simulink model "vox_ebersmoll"  (R2023b)
settings: Solver=ode1be  StartTime=0.0  StopTime=stop_time  FixedStep=Ts  RelTol=1e-3
values from neighbouring files (symbols this model uses):
  alpha_f = 236/(236+1)    (= 0.995780590717)    [dataset_generator.m]    (also in groundtruth_generator.m)
  alpha_r = 5.774/(5.774+1)    (= 0.852376734573)    [dataset_generator.m]    (also in groundtruth_generator.m)
  Is1 = 33.58e-15    (= 3.358e-14)    [dataset_generator.m]    (also in groundtruth_generator.m)
  Is2 = 33.58e-15    (= 3.358e-14)    [dataset_generator.m]    (also in groundtruth_generator.m)
  Rp1 = 1e11    (= 100000000000)    [dataset_generator.m]    (also in groundtruth_generator.m)
  Rp2 = 1e8    (= 100000000)    [dataset_generator.m]    (also in groundtruth_generator.m)
  Vt = 25.85e-3    (= 0.02585)    [dataset_generator.m]    (also in groundtruth_generator.m)
libraries: fl_lib x74, nesl_utility x11, ee_lib x1
settings Model: Creator=sebastian  LastModifiedBy=sebastian

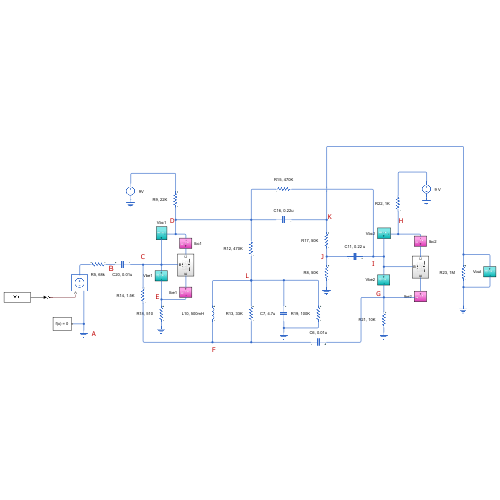
[thumbnail: Simulink's stored preview of the top-level diagram]
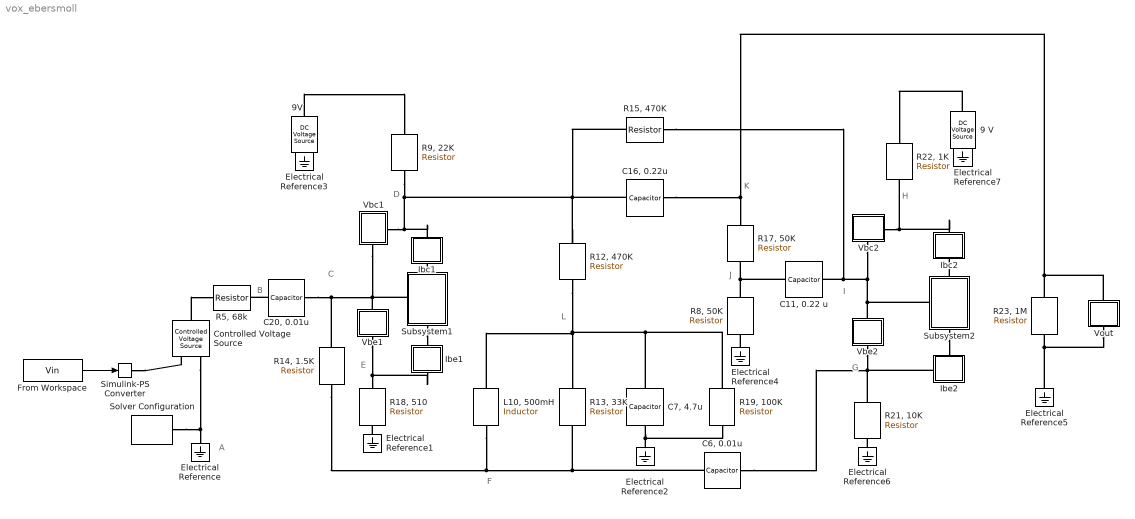
== system vox_ebersmoll ==
  note: I
  note: F
  note: E
  note: C
  note: D
  note: A
  note: B
  note: L
  note: J
  note: K
  note: G
  note: H
  9 V : fl_lib/Electrical/Electrical Sources/DC Voltage Source  v0=9 V
  9V : fl_lib/Electrical/Electrical Sources/DC Voltage Source  v0=9 V
  "C11, 0.22 u" : fl_lib/Electrical/Electrical Elements/Capacitor  c=0.22e-6 F  r=1e-6 Ohm  g=0 1/Ohm  i_specify=off  i_priority=None  i=0 A  i_nominal_specify=off  i_nominal_unit=A  i_nominal_value=1  v_specify=off  v_priority=None  v=0 V  v_nominal_specify=off  v_nominal_unit=V  v_nominal_value=1  vc_specify=off  vc_priority=High  vc=0 V  vc_nominal_specify=off  vc_nominal_unit=V  vc_nominal_value=1
  "C16, 0.22u" : fl_lib/Electrical/Electrical Elements/Capacitor  c=0.22e-6 F  r=1e-6 Ohm  g=0 1/Ohm  i_specify=off  i_priority=None  i=0 A  i_nominal_specify=off  i_nominal_unit=A  i_nominal_value=1  v_specify=off  v_priority=None  v=0 V  v_nominal_specify=off  v_nominal_unit=V  v_nominal_value=1  vc_specify=off  vc_priority=High  vc=0 V  vc_nominal_specify=off  vc_nominal_unit=V  vc_nominal_value=1
  "C20, 0.01u" : fl_lib/Electrical/Electrical Elements/Capacitor  c=0.01e-6 F  r=0 Ohm  g=0 1/Ohm  i_specify=off  i_priority=None  i=0 A  i_nominal_specify=off  i_nominal_unit=A  i_nominal_value=1  v_specify=off  v_priority=None  v=0 V  v_nominal_specify=off  v_nominal_unit=V  v_nominal_value=1  vc_specify=off  vc_priority=High  vc=0 V  vc_nominal_specify=off  vc_nominal_unit=V  vc_nominal_value=1
  "C6, 0.01u" : fl_lib/Electrical/Electrical Elements/Capacitor  c=0.01e-6 F  r=1e-6 Ohm  g=0 1/Ohm  i_specify=off  i_priority=None  i=0 A  i_nominal_specify=off  i_nominal_unit=A  i_nominal_value=1  v_specify=off  v_priority=None  v=0 V  v_nominal_specify=off  v_nominal_unit=V  v_nominal_value=1  vc_specify=off  vc_priority=High  vc=0 V  vc_nominal_specify=off  vc_nominal_unit=V  vc_nominal_value=1
  "C7, 4.7u" : fl_lib/Electrical/Electrical Elements/Capacitor  c=4.7e-6 F  r=1e-6 Ohm  g=0 1/Ohm  i_specify=off  i_priority=None  i=0 A  i_nominal_specify=off  i_nominal_unit=A  i_nominal_value=1  v_specify=off  v_priority=None  v=0 V  v_nominal_specify=off  v_nominal_unit=V  v_nominal_value=1  vc_specify=off  vc_priority=High  vc=0 V  vc_nominal_specify=off  vc_nominal_unit=V  vc_nominal_value=1
  Controlled Voltage Source : fl_lib/Electrical/Electrical Sources/Controlled Voltage Source
  Electrical Reference{,1..7} (8 alike) : fl_lib/Electrical/Electrical Elements/Electrical Reference
  From Workspace : FromWorkspace  VariableName=Vin
  Ibc1 : Subsystem
  Ibc2 : Subsystem
  Ibe1 : Subsystem
  Ibe2 : Subsystem
      settings: PortSchema="{\"entries\":[{\"content\":{\"sides\":[{\"content\":{\"connectorIds\":[\"LConn1\"]},\"type\":\"ConnectorPlacement.EquallySpacedRectSide\",\"uuid\":\"c0c77781-7d19-4b13-84c2-226c323c58f5\"},{\"content\":{\"side\":\"RIGHT\"},\"type\":\"ConnectorPlacement.EquallySpacedRectSide\",\"uuid\":\"c0907413-589c-4dc0-a622-9f77009212b7\"},{\"content\":{\"connectorIds\":[\"LConn2\"],\"side\":\"TOP\"},\"type\":\"ConnectorPlacement.EquallySpacedRectSide\",\"uuid\":\"3bc5d805-3917-4f3d-81f9-d2247414e7c8\"}]},\"type\":\"ConnectorPlacement.EquallySpacedConnector\",\"uuid\":\"4bd7f28c-fe76-4fbf-a473-c2892e027990\"}],\"packageUris\":[\"http://schema.mathworks.com/mf0/Connector/R2020b\"],\"version\":\"1.0\"}"
  "L10, 500mH" : ee_lib/Passive/Inductor  l=0.5 H  enable_L_tol=ee.enum.toleranceApplication.none  L_tol=20  tol_distribution=ee.enum.toleranceDistribution.uniform  nSigma=4  r=0 Ohm  g=1e-9 1/Ohm  enable_operating_limits=ee.enum.enable.no  operating_limit_action=ee.enum.passive.reportOpLim.warn  max_working_current=1 A  power_rating=1 W  enable_faults=ee.enum.enable.no  fault_action=simscape.enum.assert.action.none  lambdaPercent=50  k_faulted=0.9999  turnsShort=ee.enum.passive.inductor.turnsShortOption.no  openCct=ee.enum.enable.no  groundShort=ee.enum.passive.inductor.groundShortOption.no  groundShortG=0 1/Ohm  tau_fault=1e-3 s  fault_trigger=ee.enum.faults.faultTrigger.temporal  t_fault=1 s  max_permissible_voltage=100 V  n_fail_on_voltage=1  max_permissible_current=1 A  t_fail_on_current=1 s  i_L_specify=off  i_L_priority=High  i_L=0 A  i_L_nominal_specify=off  i_L_nominal_unit=A  i_L_nominal_value=1
  "R12, 470K" : fl_lib/Electrical/Electrical Elements/Resistor  R=470e3 Ohm  i_specify=off  i_priority=None  i=0 A  i_nominal_specify=off  i_nominal_unit=A  i_nominal_value=1  v_specify=off  v_priority=None  v=0 V  v_nominal_specify=off  v_nominal_unit=V  v_nominal_value=1
  "R13, 33K" : fl_lib/Electrical/Electrical Elements/Resistor  R=33e3 Ohm  i_specify=off  i_priority=None  i=0 A  i_nominal_specify=off  i_nominal_unit=A  i_nominal_value=1  v_specify=off  v_priority=None  v=0 V  v_nominal_specify=off  v_nominal_unit=V  v_nominal_value=1
  "R14, 1.5K" : fl_lib/Electrical/Electrical Elements/Resistor  R=1.5e3 Ohm  i_specify=off  i_priority=None  i=0 A  i_nominal_specify=off  i_nominal_unit=A  i_nominal_value=1  v_specify=off  v_priority=None  v=0 V  v_nominal_specify=off  v_nominal_unit=V  v_nominal_value=1
  "R15, 470K" : fl_lib/Electrical/Electrical Elements/Resistor  R=470e3 Ohm  i_specify=off  i_priority=None  i=0 A  i_nominal_specify=off  i_nominal_unit=A  i_nominal_value=1  v_specify=off  v_priority=None  v=0 V  v_nominal_specify=off  v_nominal_unit=V  v_nominal_value=1
  "R17, 50K" : fl_lib/Electrical/Electrical Elements/Resistor  R=50e3 Ohm  i_specify=off  i_priority=None  i=0 A  i_nominal_specify=off  i_nominal_unit=A  i_nominal_value=1  v_specify=off  v_priority=None  v=0 V  v_nominal_specify=off  v_nominal_unit=V  v_nominal_value=1
  "R18, 510" : fl_lib/Electrical/Electrical Elements/Resistor  R=510 Ohm  i_specify=off  i_priority=None  i=0 A  i_nominal_specify=off  i_nominal_unit=A  i_nominal_value=1  v_specify=off  v_priority=None  v=0 V  v_nominal_specify=off  v_nominal_unit=V  v_nominal_value=1
  "R19, 100K" : fl_lib/Electrical/Electrical Elements/Resistor  R=100e3 Ohm  i_specify=off  i_priority=None  i=0 A  i_nominal_specify=off  i_nominal_unit=A  i_nominal_value=1  v_specify=off  v_priority=None  v=0 V  v_nominal_specify=off  v_nominal_unit=V  v_nominal_value=1
  "R21, 10K" : fl_lib/Electrical/Electrical Elements/Resistor  R=10e3 Ohm  i_specify=off  i_priority=None  i=0 A  i_nominal_specify=off  i_nominal_unit=A  i_nominal_value=1  v_specify=off  v_priority=None  v=0 V  v_nominal_specify=off  v_nominal_unit=V  v_nominal_value=1
  "R22, 1K" : fl_lib/Electrical/Electrical Elements/Resistor  R=1e3 Ohm  i_specify=off  i_priority=None  i=0 A  i_nominal_specify=off  i_nominal_unit=A  i_nominal_value=1  v_specify=off  v_priority=None  v=0 V  v_nominal_specify=off  v_nominal_unit=V  v_nominal_value=1
  "R23, 1M" : fl_lib/Electrical/Electrical Elements/Resistor  R=1e6 Ohm  i_specify=off  i_priority=None  i=0 A  i_nominal_specify=off  i_nominal_unit=A  i_nominal_value=1  v_specify=off  v_priority=None  v=0 V  v_nominal_specify=off  v_nominal_unit=V  v_nominal_value=1
  "R5, 68k" : fl_lib/Electrical/Electrical Elements/Resistor  R=68e3 Ohm  i_specify=off  i_priority=None  i=0 A  i_nominal_specify=off  i_nominal_unit=A  i_nominal_value=1  v_specify=off  v_priority=None  v=0 V  v_nominal_specify=off  v_nominal_unit=V  v_nominal_value=1
  "R8, 50K" : fl_lib/Electrical/Electrical Elements/Resistor  R=50e3 Ohm  i_specify=off  i_priority=None  i=0 A  i_nominal_specify=off  i_nominal_unit=A  i_nominal_value=1  v_specify=off  v_priority=None  v=0 V  v_nominal_specify=off  v_nominal_unit=V  v_nominal_value=1
  "R9, 22K" : fl_lib/Electrical/Electrical Elements/Resistor  R=22e3 Ohm  i_specify=off  i_priority=None  i=0 A  i_nominal_specify=off  i_nominal_unit=A  i_nominal_value=1  v_specify=off  v_priority=None  v=0 V  v_nominal_specify=off  v_nominal_unit=V  v_nominal_value=1
  Simulink-PS Converter : nesl_utility/Simulink-PS Converter  PhysicalDomain=network_engine_domain  SubClassName=ps_input  LeftPortType=input  RightPortType=output  PseudoPeriodic=off  Frequencies=[]  NoiseDistribution=none  NoiseParameters=[]  Unit=1  AffineConversion=off  FilteringAndDerivatives=provide  SimscapeFilterOrder=1  InputFilterTimeConstant=0.001  UdotUserProvided=0
  Solver Configuration : nesl_utility/Solver Configuration  PhysicalDomain=network_engine_domain  SubClassName=solver  LeftPortType=input  RightPortType=generic  Tones=[]  Harmonics=[]  SimulateNoise=off  Profile=off  UseLocalSampling=off  EnableSwitchedLinearOptims=on  FrequencyDomain=off  UseCCode=off  RelTol=0.001  AbsTol=0.001  MinStep=1e-09  ToWorkspace=off  RevertToSquareIcSolve=off  NumHomotopyIterations=100  PhasorMode=off  PhasorModeNumHarmonics=1  ConsistencySolver=NEWTON_XTOL_AFTER_FTOL  IndexReductionMethod=DerivativeReplacement  DoDC=on  ResidualTolerance=1e-09  ConsistencyTolSource=GLOBAL  ConsistencyAbsTol=0.001  ConsistencyRelTol=0.001  ConsistencyTolFactor=0.001  UseLocalSolver=off  LocalSolverChoice=NE_BACKWARD_EULER_ADVANCER  ResolveIndetEquations=on  FunctionEvalNumThread=1  LocalSolverSampleTime=0.001  DoFixedCost=off  MaxNonlinIter=3  MaxModeIter=2  ComputeImpulses=off  ImpulseIterations=2  LinearAlgebra=auto  LinearAlgebraNumThread=0  EquationFormulation=NE_TIME_EF  DelaysMemoryBudget=1024  AutomaticFiltering=on  FilteringTimeConstant=0.001  PartitionStorageMethod=AS_NEEDED  PartitionMemoryBudget=1024  PartitionMethod=ROBUST  MultibodyUseLocalSolver=off  MultibodyLocalSolverChoice=ODE1  MultibodyLocalSolverSampleTime=0.001
  Subsystem1 : Subsystem
      settings: PortSchema="{\"entries\":[{\"content\":{\"sides\":[{\"content\":{\"connectorIds\":[\"LConn1\"]},\"type\":\"ConnectorPlacement.EquallySpacedRectSide\",\"uuid\":\"e7d2ad01-b729-4278-a2af-615928332c77\"},{\"content\":{\"side\":\"RIGHT\"},\"type\":\"ConnectorPlacement.EquallySpacedRectSide\",\"uuid\":\"6c8f5083-1d74-476b-8fc8-74f7e6a90163\"},{\"content\":{\"connectorIds\":[\"LConn2\"],\"side\":\"TOP\"},\"type\":\"ConnectorPlacement.EquallySpacedRectSide\",\"uuid\":\"cf8d2faf-1e25-415e-bca0-3701d5262d4d\"},{\"content\":{\"connectorIds\":[\"RConn1\"],\"side\":\"BOTTOM\"},\"type\":\"ConnectorPlacement.EquallySpacedRectSide\",\"uuid\":\"80ad8aee-c458-4554-96ef-dc25eb201335\"}]},\"type\":\"ConnectorPlacement.EquallySpacedConnector\",\"uuid\":\"23596b54-1579-47cb-b7ec-00e276fa3e81\"}],\"packageUris\":[\"http://schema.mathworks.com/mf0/Connector/R2020b\"],\"version\":\"1.0\"}"
  Subsystem2 : Subsystem
      settings: PortSchema="{\"entries\":[{\"content\":{\"sides\":[{\"content\":{\"connectorIds\":[\"LConn1\"]},\"type\":\"ConnectorPlacement.EquallySpacedRectSide\",\"uuid\":\"e7d2ad01-b729-4278-a2af-615928332c77\"},{\"content\":{\"side\":\"RIGHT\"},\"type\":\"ConnectorPlacement.EquallySpacedRectSide\",\"uuid\":\"6c8f5083-1d74-476b-8fc8-74f7e6a90163\"},{\"content\":{\"connectorIds\":[\"LConn2\"],\"side\":\"TOP\"},\"type\":\"ConnectorPlacement.EquallySpacedRectSide\",\"uuid\":\"cf8d2faf-1e25-415e-bca0-3701d5262d4d\"},{\"content\":{\"connectorIds\":[\"RConn1\"],\"side\":\"BOTTOM\"},\"type\":\"ConnectorPlacement.EquallySpacedRectSide\",\"uuid\":\"80ad8aee-c458-4554-96ef-dc25eb201335\"}]},\"type\":\"ConnectorPlacement.EquallySpacedConnector\",\"uuid\":\"23596b54-1579-47cb-b7ec-00e276fa3e81\"}],\"packageUris\":[\"http://schema.mathworks.com/mf0/Connector/R2020b\"],\"version\":\"1.0\"}"
  Vbc1 : Subsystem
      settings: PortSchema="{\"entries\":[{\"content\":{\"sides\":[{\"content\":{\"connectorIds\":[\"LConn1\"]},\"type\":\"ConnectorPlacement.EquallySpacedRectSide\",\"uuid\":\"7eb44552-7f97-4ce7-929d-c8e8969a6339\"},{\"content\":{\"side\":\"RIGHT\"},\"type\":\"ConnectorPlacement.EquallySpacedRectSide\",\"uuid\":\"ace6a3d5-1573-4a81-b16e-bbe1b3c73136\"},{\"content\":{\"side\":\"TOP\"},\"type\":\"ConnectorPlacement.EquallySpacedRectSide\",\"uuid\":\"f287eb84-5a92-47a0-b0c0-f16ac8f6c1fa\"},{\"content\":{\"connectorIds\":[\"RConn1\"],\"side\":\"BOTTOM\"},\"type\":\"ConnectorPlacement.EquallySpacedRectSide\",\"uuid\":\"ef144dba-d688-4ec6-a3ad-e1b4e02b5e22\"}]},\"type\":\"ConnectorPlacement.EquallySpacedConnector\",\"uuid\":\"265b9e65-e5e0-4894-94ad-1de7b98f8ce0\"}],\"packageUris\":[\"http://schema.mathworks.com/mf0/Connector/R2020b\"],\"version\":\"1.0\"}"
  Vbc2 : Subsystem
      settings: PortSchema="{\"entries\":[{\"content\":{\"sides\":[{\"content\":{},\"type\":\"ConnectorPlacement.EquallySpacedRectSide\",\"uuid\":\"7eb44552-7f97-4ce7-929d-c8e8969a6339\"},{\"content\":{\"connectorIds\":[\"RConn1\"],\"side\":\"RIGHT\"},\"type\":\"ConnectorPlacement.EquallySpacedRectSide\",\"uuid\":\"ace6a3d5-1573-4a81-b16e-bbe1b3c73136\"},{\"content\":{\"side\":\"TOP\"},\"type\":\"ConnectorPlacement.EquallySpacedRectSide\",\"uuid\":\"f287eb84-5a92-47a0-b0c0-f16ac8f6c1fa\"},{\"content\":{\"connectorIds\":[\"RConn2\"],\"side\":\"BOTTOM\"},\"type\":\"ConnectorPlacement.EquallySpacedRectSide\",\"uuid\":\"ef144dba-d688-4ec6-a3ad-e1b4e02b5e22\"}]},\"type\":\"ConnectorPlacement.EquallySpacedConnector\",\"uuid\":\"265b9e65-e5e0-4894-94ad-1de7b98f8ce0\"}],\"packageUris\":[\"http://schema.mathworks.com/mf0/Connector/R2020b\"],\"version\":\"1.0\"}"
  Vbe1 : Subsystem
  Vbe2 : Subsystem
  Vout : Subsystem
  wires:
  From Workspace/1 -> Simulink-PS Converter/1
  connections:
  Solver Configuration/RConn1 -- Controlled Voltage Source/RConn2 -- Electrical Reference/LConn1
  Controlled Voltage Source/LConn1 -- "R5, 68k"/LConn1
  "C20, 0.01u"/LConn1 -- "R5, 68k"/RConn1
  "R9, 22K"/RConn1 -- Vbc1/LConn1 -- Ibc1/RConn1 -- "R15, 470K"/RConn1 -- "R12, 470K"/LConn1 -- "C16, 0.22u"/RConn1
  Electrical Reference3/LConn1 -- 9V/RConn1
  Vbe1/LConn1 -- Vbc1/RConn1 -- "C20, 0.01u"/RConn1 -- "R14, 1.5K"/LConn1 -- Subsystem1/LConn1
  Vbe1/RConn1 -- Ibe1/RConn1 -- "R18, 510"/LConn1
  "R12, 470K"/RConn1 -- "R13, 33K"/LConn1 -- "L10, 500mH"/LConn1 -- "R19, 100K"/LConn1 -- "C7, 4.7u"/LConn1
  "L10, 500mH"/RConn1 -- "R14, 1.5K"/RConn1 -- "C6, 0.01u"/RConn1 -- "R13, 33K"/RConn1
  Electrical Reference2/LConn1 -- "R19, 100K"/RConn1 -- "C7, 4.7u"/RConn1
  "R8, 50K"/LConn1 -- "C11, 0.22 u"/RConn1 -- "R17, 50K"/RConn1
  "C16, 0.22u"/LConn1 -- Vout/LConn1 -- "R23, 1M"/LConn1 -- "R17, 50K"/LConn1
  Electrical Reference4/LConn1 -- "R8, 50K"/RConn1
  "R15, 470K"/LConn1 -- Vbe2/LConn1 -- Subsystem2/LConn1 -- Vbc2/RConn1 -- "C11, 0.22 u"/LConn1
  Electrical Reference5/LConn1 -- Vout/RConn1 -- "R23, 1M"/RConn1
  "C6, 0.01u"/LConn1 -- Ibe2/LConn2 -- "R21, 10K"/LConn1 -- Vbe2/RConn1
  Electrical Reference6/LConn1 -- "R21, 10K"/RConn1
  Vbc2/RConn2 -- Ibc2/RConn1 -- "R22, 1K"/RConn1
  Electrical Reference7/LConn1 -- 9 V/RConn1
  9 V/LConn1 -- "R22, 1K"/LConn1
  Simulink-PS Converter/RConn1 -- Controlled Voltage Source/RConn1
  Subsystem1/RConn1 -- Ibe1/LConn1
  Subsystem1/LConn2 -- Ibc1/LConn1
  Subsystem2/LConn2 -- Ibc2/LConn1
  Subsystem2/RConn1 -- Ibe2/LConn1
  9V/LConn1 -- "R9, 22K"/LConn1
  Electrical Reference1/LConn1 -- "R18, 510"/RConn1

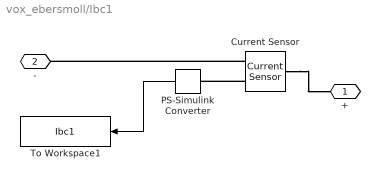
== system vox_ebersmoll/Ibc1 ==
  Current Sensor : fl_lib/Electrical/Electrical Sensors/Current Sensor
  PS-Simulink Converter : nesl_utility/PS-Simulink Converter  PhysicalDomain=network_engine_domain  SubClassName=ps_output  LeftPortType=input  RightPortType=output  PseudoPeriodic=off  Frequencies=[]  VectorFormat=1-D array  Unit=1  AffineConversion=off
  To Workspace1 : ToWorkspace  VariableName=Ibc1  SaveFormat=Timeseries  SampleTime=-1
  + : PMIOPort  Side=Left
  - : PMIOPort  Port=2  Side=Right
  wires:
  PS-Simulink Converter/1 -> To Workspace1/1
  connections:
  Current Sensor/RConn2 -- -/RConn1
  Current Sensor/RConn1 -- PS-Simulink Converter/LConn1
  Current Sensor/LConn1 -- +/RConn1

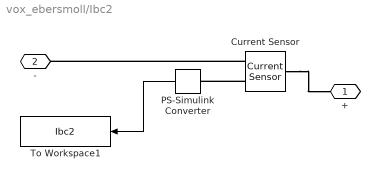
== system vox_ebersmoll/Ibc2 ==
  Current Sensor : fl_lib/Electrical/Electrical Sensors/Current Sensor
  PS-Simulink Converter : nesl_utility/PS-Simulink Converter  PhysicalDomain=network_engine_domain  SubClassName=ps_output  LeftPortType=input  RightPortType=output  PseudoPeriodic=off  Frequencies=[]  VectorFormat=1-D array  Unit=1  AffineConversion=off
  To Workspace1 : ToWorkspace  VariableName=Ibc2  SaveFormat=Timeseries  SampleTime=-1
  + : PMIOPort  Side=Left
  - : PMIOPort  Port=2  Side=Right
  wires:
  PS-Simulink Converter/1 -> To Workspace1/1
  connections:
  Current Sensor/RConn2 -- -/RConn1
  Current Sensor/RConn1 -- PS-Simulink Converter/LConn1
  Current Sensor/LConn1 -- +/RConn1

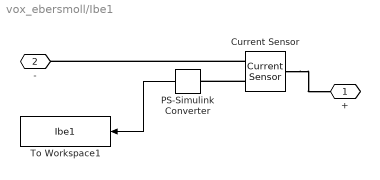
== system vox_ebersmoll/Ibe1 ==
  Current Sensor : fl_lib/Electrical/Electrical Sensors/Current Sensor
  PS-Simulink Converter : nesl_utility/PS-Simulink Converter  PhysicalDomain=network_engine_domain  SubClassName=ps_output  LeftPortType=input  RightPortType=output  PseudoPeriodic=off  Frequencies=[]  VectorFormat=1-D array  Unit=1  AffineConversion=off
  To Workspace1 : ToWorkspace  VariableName=Ibe1  SaveFormat=Timeseries  SampleTime=-1
  + : PMIOPort  Side=Left
  - : PMIOPort  Port=2  Side=Right
  wires:
  PS-Simulink Converter/1 -> To Workspace1/1
  connections:
  Current Sensor/RConn2 -- -/RConn1
  Current Sensor/RConn1 -- PS-Simulink Converter/LConn1
  Current Sensor/LConn1 -- +/RConn1

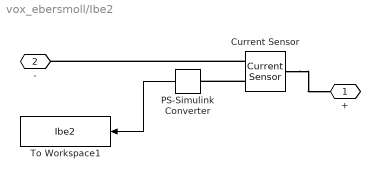
== system vox_ebersmoll/Ibe2 ==
  Current Sensor : fl_lib/Electrical/Electrical Sensors/Current Sensor
  PS-Simulink Converter : nesl_utility/PS-Simulink Converter  PhysicalDomain=network_engine_domain  SubClassName=ps_output  LeftPortType=input  RightPortType=output  PseudoPeriodic=off  Frequencies=[]  VectorFormat=1-D array  Unit=1  AffineConversion=off
  To Workspace1 : ToWorkspace  VariableName=Ibe2  SaveFormat=Timeseries  SampleTime=-1
  + : PMIOPort  Side=Left
  - : PMIOPort  Port=2  Side=Left
  wires:
  PS-Simulink Converter/1 -> To Workspace1/1
  connections:
  Current Sensor/RConn2 -- -/RConn1
  Current Sensor/RConn1 -- PS-Simulink Converter/LConn1
  Current Sensor/LConn1 -- +/RConn1

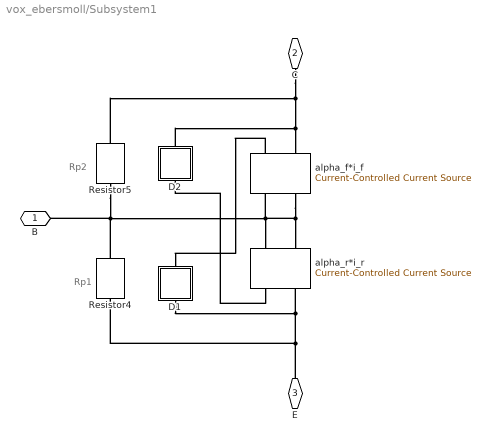
== system vox_ebersmoll/Subsystem1 ==
  note: Rp1
  note: Rp2
  D1 : Subsystem
  D2 : Subsystem
  Resistor4 : fl_lib/Electrical/Electrical Elements/Resistor  R=Rp1 Ohm  i_specify=off  i_priority=None  i=0 A  i_nominal_specify=off  i_nominal_unit=A  i_nominal_value=1  v_specify=off  v_priority=None  v=0 V  v_nominal_specify=off  v_nominal_unit=V  v_nominal_value=1
  Resistor5 : fl_lib/Electrical/Electrical Elements/Resistor  R=Rp2 Ohm  i_specify=off  i_priority=None  i=0 A  i_nominal_specify=off  i_nominal_unit=A  i_nominal_value=1  v_specify=off  v_priority=None  v=0 V  v_nominal_specify=off  v_nominal_unit=V  v_nominal_value=1
  alpha_f*i_f : fl_lib/Electrical/Electrical Sources/Current-Controlled Current Source  K=alpha_f  i1_specify=off  i1_priority=High  i1=0 A  i1_nominal_specify=off  i1_nominal_unit=A  i1_nominal_value=1  i2_specify=off  i2_priority=High  i2=0 A  i2_nominal_specify=off  i2_nominal_unit=A  i2_nominal_value=1
      settings: InternalSimscapePortConfiguration="{\"Bottom\":[],\"Left\":[{\"id\":\"p1\",\"label\":\"+\",\"type\":\"foundation.electrical.electrical\"},{\"id\":\"head\",\"label\":\"\",\"type\":\"foundation.electrical.electrical\"}],\"Right\":[{\"id\":\"n1\",\"label\":\"-\",\"type\":\"foundation.electrical.electrical\"},{\"id\":\"tail\",\"label\":\"\",\"type\":\"foundation.electrical.electrical\"}],\"Top\":[]}"
  alpha_r*i_r : fl_lib/Electrical/Electrical Sources/Current-Controlled Current Source  K=alpha_r  i1_specify=off  i1_priority=High  i1=0 A  i1_nominal_specify=off  i1_nominal_unit=A  i1_nominal_value=1  i2_specify=off  i2_priority=High  i2=0 A  i2_nominal_specify=off  i2_nominal_unit=A  i2_nominal_value=1
      settings: InternalSimscapePortConfiguration="{\"Bottom\":[],\"Left\":[{\"id\":\"p1\",\"label\":\"+\",\"type\":\"foundation.electrical.electrical\"},{\"id\":\"head\",\"label\":\"\",\"type\":\"foundation.electrical.electrical\"}],\"Right\":[{\"id\":\"n1\",\"label\":\"-\",\"type\":\"foundation.electrical.electrical\"},{\"id\":\"tail\",\"label\":\"\",\"type\":\"foundation.electrical.electrical\"}],\"Top\":[]}"
  B : PMIOPort  Side=Left
  C : PMIOPort  Port=2  Side=Left
  E : PMIOPort  Port=3  Side=Right
  connections:
  D1/RConn1 -- alpha_r*i_r/RConn2 -- E/RConn1 -- Resistor4/RConn1
  D2/RConn1 -- alpha_f*i_f/RConn2 -- C/RConn1 -- Resistor5/LConn1
  alpha_f*i_f/LConn1 -- alpha_r*i_r/LConn1 -- alpha_r*i_r/LConn2 -- alpha_f*i_f/LConn2 -- Resistor4/LConn1 -- B/RConn1 -- Resistor5/RConn1
  alpha_f*i_f/RConn1 -- D1/LConn1
  alpha_r*i_r/RConn1 -- D2/LConn1

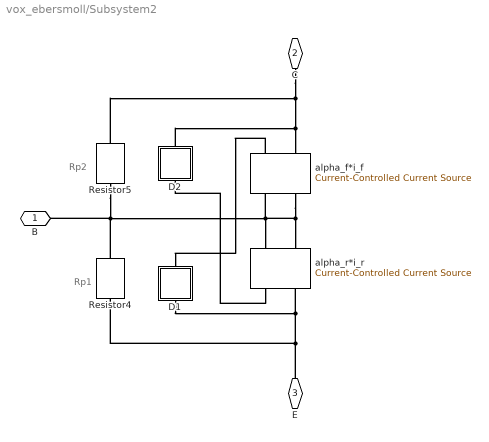
== system vox_ebersmoll/Subsystem2 ==
  note: Rp1
  note: Rp2
  D1 : Subsystem
  D2 : Subsystem
  Resistor4 : fl_lib/Electrical/Electrical Elements/Resistor  R=Rp1 Ohm  i_specify=off  i_priority=None  i=0 A  i_nominal_specify=off  i_nominal_unit=A  i_nominal_value=1  v_specify=off  v_priority=None  v=0 V  v_nominal_specify=off  v_nominal_unit=V  v_nominal_value=1
  Resistor5 : fl_lib/Electrical/Electrical Elements/Resistor  R=Rp2 Ohm  i_specify=off  i_priority=None  i=0 A  i_nominal_specify=off  i_nominal_unit=A  i_nominal_value=1  v_specify=off  v_priority=None  v=0 V  v_nominal_specify=off  v_nominal_unit=V  v_nominal_value=1
  alpha_f*i_f : fl_lib/Electrical/Electrical Sources/Current-Controlled Current Source  K=alpha_f  i1_specify=off  i1_priority=High  i1=0 A  i1_nominal_specify=off  i1_nominal_unit=A  i1_nominal_value=1  i2_specify=off  i2_priority=High  i2=0 A  i2_nominal_specify=off  i2_nominal_unit=A  i2_nominal_value=1
      settings: InternalSimscapePortConfiguration="{\"Bottom\":[],\"Left\":[{\"id\":\"p1\",\"label\":\"+\",\"type\":\"foundation.electrical.electrical\"},{\"id\":\"head\",\"label\":\"\",\"type\":\"foundation.electrical.electrical\"}],\"Right\":[{\"id\":\"n1\",\"label\":\"-\",\"type\":\"foundation.electrical.electrical\"},{\"id\":\"tail\",\"label\":\"\",\"type\":\"foundation.electrical.electrical\"}],\"Top\":[]}"
  alpha_r*i_r : fl_lib/Electrical/Electrical Sources/Current-Controlled Current Source  K=alpha_r  i1_specify=off  i1_priority=High  i1=0 A  i1_nominal_specify=off  i1_nominal_unit=A  i1_nominal_value=1  i2_specify=off  i2_priority=High  i2=0 A  i2_nominal_specify=off  i2_nominal_unit=A  i2_nominal_value=1
      settings: InternalSimscapePortConfiguration="{\"Bottom\":[],\"Left\":[{\"id\":\"p1\",\"label\":\"+\",\"type\":\"foundation.electrical.electrical\"},{\"id\":\"head\",\"label\":\"\",\"type\":\"foundation.electrical.electrical\"}],\"Right\":[{\"id\":\"n1\",\"label\":\"-\",\"type\":\"foundation.electrical.electrical\"},{\"id\":\"tail\",\"label\":\"\",\"type\":\"foundation.electrical.electrical\"}],\"Top\":[]}"
  B : PMIOPort  Side=Left
  C : PMIOPort  Port=2  Side=Left
  E : PMIOPort  Port=3  Side=Right
  connections:
  D1/RConn1 -- alpha_r*i_r/RConn2 -- E/RConn1 -- Resistor4/RConn1
  D2/RConn1 -- alpha_f*i_f/RConn2 -- C/RConn1 -- Resistor5/LConn1
  alpha_f*i_f/LConn1 -- alpha_r*i_r/LConn1 -- alpha_r*i_r/LConn2 -- alpha_f*i_f/LConn2 -- Resistor4/LConn1 -- B/RConn1 -- Resistor5/RConn1
  alpha_f*i_f/RConn1 -- D1/LConn1
  alpha_r*i_r/RConn1 -- D2/LConn1

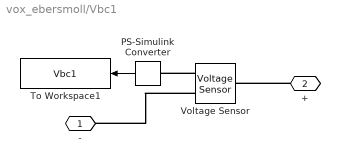
== system vox_ebersmoll/Vbc1 ==
  PS-Simulink Converter : nesl_utility/PS-Simulink Converter  PhysicalDomain=network_engine_domain  SubClassName=ps_output  LeftPortType=input  RightPortType=output  PseudoPeriodic=off  Frequencies=[]  VectorFormat=1-D array  Unit=1  AffineConversion=off
  To Workspace1 : ToWorkspace  VariableName=Vbc1  SaveFormat=Timeseries  SampleTime=-1
  Voltage Sensor : fl_lib/Electrical/Electrical Sensors/Voltage Sensor
  - : PMIOPort  Side=Left
  + : PMIOPort  Port=2  Side=Right
  wires:
  PS-Simulink Converter/1 -> To Workspace1/1
  connections:
  Voltage Sensor/RConn2 -- -/RConn1
  Voltage Sensor/RConn1 -- PS-Simulink Converter/LConn1
  +/RConn1 -- Voltage Sensor/LConn1

== system vox_ebersmoll/Vbc2 ==
  PS-Simulink Converter : nesl_utility/PS-Simulink Converter  PhysicalDomain=network_engine_domain  SubClassName=ps_output  LeftPortType=input  RightPortType=output  PseudoPeriodic=off  Frequencies=[]  VectorFormat=1-D array  Unit=1  AffineConversion=off
  To Workspace1 : ToWorkspace  VariableName=Vbc2  SaveFormat=Timeseries  SampleTime=-1
  Voltage Sensor : fl_lib/Electrical/Electrical Sensors/Voltage Sensor
  + : PMIOPort  Side=Right
  - : PMIOPort  Port=2  Side=Right
  wires:
  PS-Simulink Converter/1 -> To Workspace1/1
  connections:
  Voltage Sensor/RConn2 -- -/RConn1
  Voltage Sensor/RConn1 -- PS-Simulink Converter/LConn1
  +/RConn1 -- Voltage Sensor/LConn1

== system vox_ebersmoll/Vbe1 ==
  PS-Simulink Converter : nesl_utility/PS-Simulink Converter  PhysicalDomain=network_engine_domain  SubClassName=ps_output  LeftPortType=input  RightPortType=output  PseudoPeriodic=off  Frequencies=[]  VectorFormat=1-D array  Unit=1  AffineConversion=off
  To Workspace1 : ToWorkspace  VariableName=Vbe1  SaveFormat=Timeseries  SampleTime=-1
  Voltage Sensor : fl_lib/Electrical/Electrical Sensors/Voltage Sensor
  + : PMIOPort  Side=Left
  - : PMIOPort  Port=2  Side=Right
  wires:
  PS-Simulink Converter/1 -> To Workspace1/1
  connections:
  Voltage Sensor/RConn2 -- -/RConn1
  Voltage Sensor/RConn1 -- PS-Simulink Converter/LConn1
  +/RConn1 -- Voltage Sensor/LConn1

== system vox_ebersmoll/Vbe2 ==
  PS-Simulink Converter : nesl_utility/PS-Simulink Converter  PhysicalDomain=network_engine_domain  SubClassName=ps_output  LeftPortType=input  RightPortType=output  PseudoPeriodic=off  Frequencies=[]  VectorFormat=1-D array  Unit=1  AffineConversion=off
  To Workspace1 : ToWorkspace  VariableName=Vbe2  SaveFormat=Timeseries  SampleTime=-1
  Voltage Sensor : fl_lib/Electrical/Electrical Sensors/Voltage Sensor
  + : PMIOPort  Side=Left
  - : PMIOPort  Port=2  Side=Right
  wires:
  PS-Simulink Converter/1 -> To Workspace1/1
  connections:
  Voltage Sensor/RConn2 -- -/RConn1
  Voltage Sensor/RConn1 -- PS-Simulink Converter/LConn1
  +/RConn1 -- Voltage Sensor/LConn1

== system vox_ebersmoll/Vout ==
  PS-Simulink Converter : nesl_utility/PS-Simulink Converter  PhysicalDomain=network_engine_domain  SubClassName=ps_output  LeftPortType=input  RightPortType=output  PseudoPeriodic=off  Frequencies=[]  VectorFormat=1-D array  Unit=1  AffineConversion=off
  To Workspace1 : ToWorkspace  VariableName=Vout  SaveFormat=Timeseries  SampleTime=-1
  Voltage Sensor : fl_lib/Electrical/Electrical Sensors/Voltage Sensor
  + : PMIOPort  Side=Left
  - : PMIOPort  Port=2  Side=Right
  wires:
  PS-Simulink Converter/1 -> To Workspace1/1
  connections:
  Voltage Sensor/RConn2 -- -/RConn1
  Voltage Sensor/RConn1 -- PS-Simulink Converter/LConn1
  +/RConn1 -- Voltage Sensor/LConn1

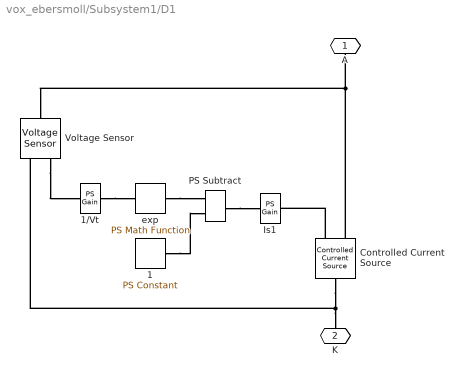
== system vox_ebersmoll/Subsystem1/D1 ==
  1 : fl_lib/Physical Signals/Sources/PS Constant  constant=1
  1/Vt : fl_lib/Physical Signals/Functions/PS Gain  gain=1/Vt 1/V
  Controlled Current Source : fl_lib/Electrical/Electrical Sources/Controlled Current Source
  Is1 : fl_lib/Physical Signals/Functions/PS Gain  gain=Is1 A
  PS Subtract : fl_lib/Physical Signals/Functions/PS Subtract
  Voltage Sensor : fl_lib/Electrical/Electrical Sensors/Voltage Sensor
  exp : fl_lib/Physical Signals/Functions/PS Math Function  fcn_choice=3  v=1
  A : PMIOPort  Side=Left
  K : PMIOPort  Port=2  Side=Right
  connections:
  K/RConn1 -- Controlled Current Source/LConn1 -- Voltage Sensor/RConn2
  Controlled Current Source/RConn1 -- Is1/RConn1
  PS Subtract/RConn1 -- Is1/LConn1
  1/RConn1 -- PS Subtract/LConn2
  exp/RConn1 -- PS Subtract/LConn1
  1/Vt/RConn1 -- exp/LConn1
  Voltage Sensor/RConn1 -- 1/Vt/LConn1
  A/RConn1 -- Voltage Sensor/LConn1 -- Controlled Current Source/RConn2

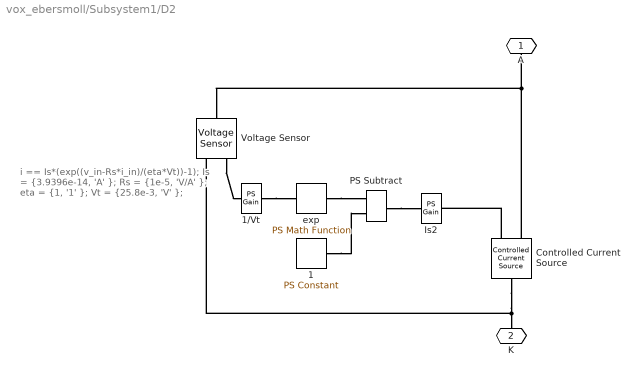
== system vox_ebersmoll/Subsystem1/D2 ==
  note: i == Is*(exp((v_in-Rs*i_in)/(eta*Vt))-1);
      | Is = {3.9396e-14, 'A' };
      | Rs = {1e-5, 'V/A' };
      | eta = {1, '1' };
      | Vt = {25.8e-3, 'V' };
  1 : fl_lib/Physical Signals/Sources/PS Constant  constant=1
  1/Vt : fl_lib/Physical Signals/Functions/PS Gain  gain=1/Vt 1/V
  Controlled Current Source : fl_lib/Electrical/Electrical Sources/Controlled Current Source
  Is2 : fl_lib/Physical Signals/Functions/PS Gain  gain=Is2 A
  PS Subtract : fl_lib/Physical Signals/Functions/PS Subtract
  Voltage Sensor : fl_lib/Electrical/Electrical Sensors/Voltage Sensor
  exp : fl_lib/Physical Signals/Functions/PS Math Function  fcn_choice=3  v=1
  A : PMIOPort  Side=Left
  K : PMIOPort  Port=2  Side=Right
  connections:
  Controlled Current Source/RConn2 -- Voltage Sensor/LConn1 -- A/RConn1
  Voltage Sensor/RConn1 -- 1/Vt/LConn1
  1/Vt/RConn1 -- exp/LConn1
  exp/RConn1 -- PS Subtract/LConn1
  1/RConn1 -- PS Subtract/LConn2
  PS Subtract/RConn1 -- Is2/LConn1
  Controlled Current Source/RConn1 -- Is2/RConn1
  K/RConn1 -- Voltage Sensor/RConn2 -- Controlled Current Source/LConn1

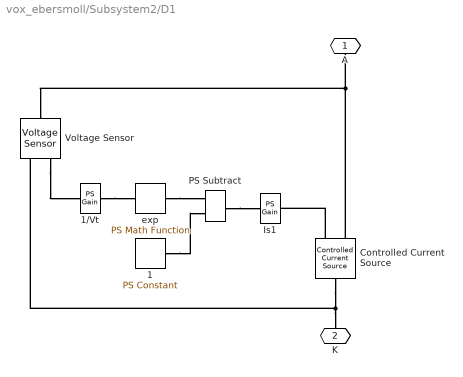
== system vox_ebersmoll/Subsystem2/D1 ==
  1 : fl_lib/Physical Signals/Sources/PS Constant  constant=1
  1/Vt : fl_lib/Physical Signals/Functions/PS Gain  gain=1/Vt 1/V
  Controlled Current Source : fl_lib/Electrical/Electrical Sources/Controlled Current Source
  Is1 : fl_lib/Physical Signals/Functions/PS Gain  gain=Is1 A
  PS Subtract : fl_lib/Physical Signals/Functions/PS Subtract
  Voltage Sensor : fl_lib/Electrical/Electrical Sensors/Voltage Sensor
  exp : fl_lib/Physical Signals/Functions/PS Math Function  fcn_choice=3  v=1
  A : PMIOPort  Side=Left
  K : PMIOPort  Port=2  Side=Right
  connections:
  K/RConn1 -- Controlled Current Source/LConn1 -- Voltage Sensor/RConn2
  Controlled Current Source/RConn1 -- Is1/RConn1
  PS Subtract/RConn1 -- Is1/LConn1
  1/RConn1 -- PS Subtract/LConn2
  exp/RConn1 -- PS Subtract/LConn1
  1/Vt/RConn1 -- exp/LConn1
  Voltage Sensor/RConn1 -- 1/Vt/LConn1
  A/RConn1 -- Voltage Sensor/LConn1 -- Controlled Current Source/RConn2

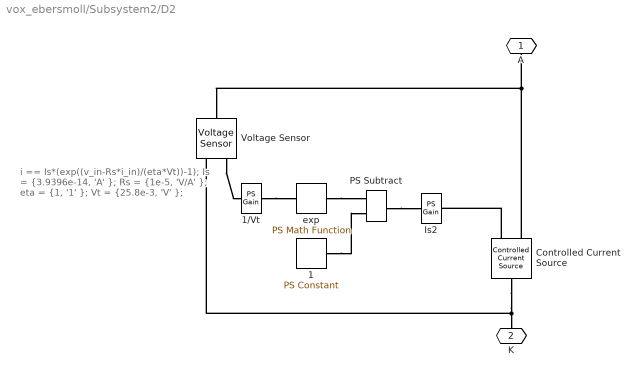
== system vox_ebersmoll/Subsystem2/D2 ==
  note: i == Is*(exp((v_in-Rs*i_in)/(eta*Vt))-1);
      | Is = {3.9396e-14, 'A' };
      | Rs = {1e-5, 'V/A' };
      | eta = {1, '1' };
      | Vt = {25.8e-3, 'V' };
  1 : fl_lib/Physical Signals/Sources/PS Constant  constant=1
  1/Vt : fl_lib/Physical Signals/Functions/PS Gain  gain=1/Vt 1/V
  Controlled Current Source : fl_lib/Electrical/Electrical Sources/Controlled Current Source
  Is2 : fl_lib/Physical Signals/Functions/PS Gain  gain=Is2 A
  PS Subtract : fl_lib/Physical Signals/Functions/PS Subtract
  Voltage Sensor : fl_lib/Electrical/Electrical Sensors/Voltage Sensor
  exp : fl_lib/Physical Signals/Functions/PS Math Function  fcn_choice=3  v=1
  A : PMIOPort  Side=Left
  K : PMIOPort  Port=2  Side=Right
  connections:
  Controlled Current Source/RConn2 -- Voltage Sensor/LConn1 -- A/RConn1
  Voltage Sensor/RConn1 -- 1/Vt/LConn1
  1/Vt/RConn1 -- exp/LConn1
  exp/RConn1 -- PS Subtract/LConn1
  1/RConn1 -- PS Subtract/LConn2
  PS Subtract/RConn1 -- Is2/LConn1
  Controlled Current Source/RConn1 -- Is2/RConn1
  K/RConn1 -- Voltage Sensor/RConn2 -- Controlled Current Source/LConn1
